simulink model "modeloNL1_HIL"  (R2025a)
settings: Solver=ode4  StartTime=0.0  StopTime=30  FixedStep=0.01  RelTol=1e-3
settings Model: Creator=anade  LastModifiedBy=Kaue

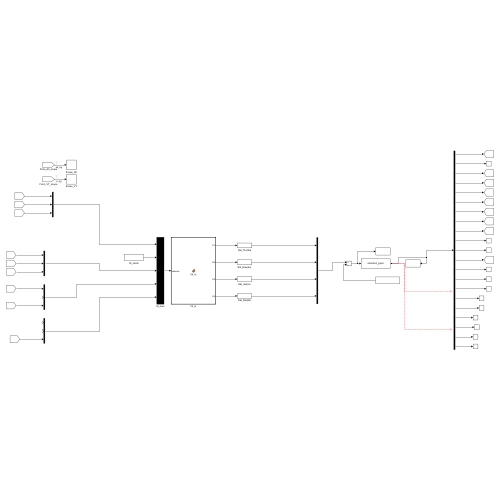
[thumbnail: Simulink's stored preview of the top-level diagram]
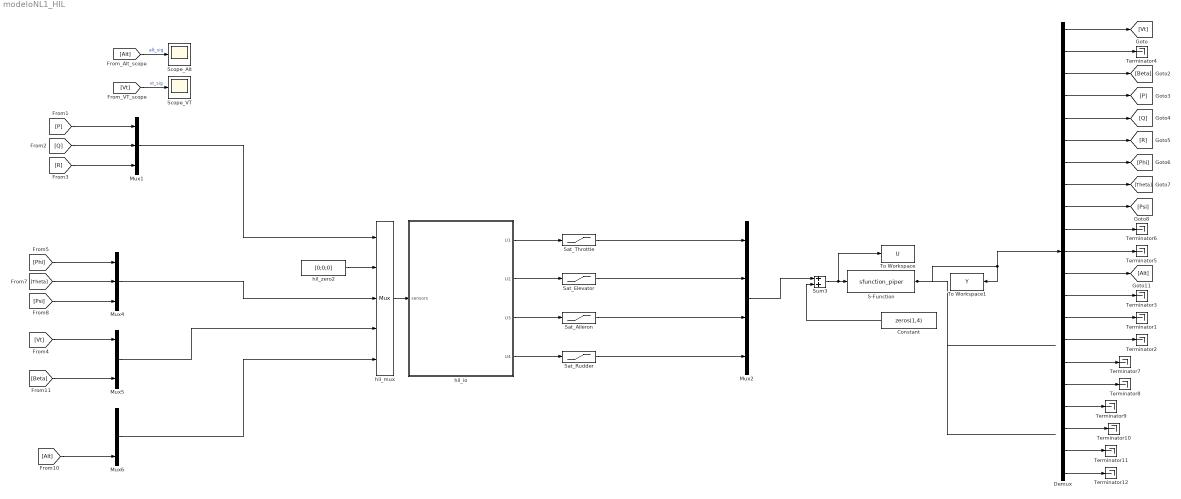
== system modeloNL1_HIL ==
  Constant : Constant  Value=zeros(1,4)
  Demux : Demux  Outputs=21
  Mux{1,4..6} (4 alike) : Mux  Inputs=3
  Mux2 : Mux
  S-Function : S-Function  FunctionName=sfunction_piper  Parameters=par_gen,par_aero,par_prop, Xe  SFunctionDeploymentMode=off  EnableBusSupport=off
  Sat_Aileron : Saturate  UpperLimit=0.4363  LowerLimit=-0.4363
  Sat_Elevator : Saturate  UpperLimit=0.4363  LowerLimit=-0.4363
  Sat_Rudder : Saturate  UpperLimit=0.4363  LowerLimit=-0.4363
  Sat_Throttle : Saturate  UpperLimit=1  LowerLimit=0
  Scope_Alt : Scope
      settings: ActiveDisplayYMinimum=80  ActiveDisplayYMaximum=120
  Scope_VT : Scope
      settings: ActiveDisplayYMinimum=10  ActiveDisplayYMaximum=20
  Sum3 : Sum
  Terminator{1..12} (12 alike) : Terminator
  To Workspace : ToWorkspace  VariableName=U  SaveFormat=Structure With Time  SampleTime=-1
  To Workspace1 : ToWorkspace  VariableName=Y  SaveFormat=Structure With Time  SampleTime=-1
  hil_io : MATLAB Function  TreatAsAtomicUnit=on
  hil_mux : Mux  Inputs=5
  hil_zero2 : Constant  Value=[0;0;0]
  wires:
  S-Function/1 -> To Workspace1/1, Demux/1
  Sum3/1 -> To Workspace/1, S-Function/1
  Mux2/1 -> Sum3/1
  Constant/1 -> Sum3/2
  Demux/2 -> Terminator4/1
  Demux/3 -> [Beta]
  Demux/4 -> [P]
  Demux/5 -> [Q]
  Demux/6 -> [R]
  Demux/7 -> [Phi]
  Demux/8 -> [Theta]
  Demux/10 -> Terminator6/1
  Demux/11 -> Terminator5/1
  Demux/13 -> Terminator3/1
  Demux/14 -> Terminator1/1
  Demux/15 -> Terminator2/1
  Demux/1 -> [Vt]
  [Theta] -> Mux4/2
  Mux1/1 -> hil_mux/1
  [Alt] -> Mux6/3
  [P] -> Mux1/1
  Mux4/1 -> hil_mux/3
  [R] -> Mux1/3
  [Phi] -> Mux4/1
  Mux6/1 -> hil_mux/5
  [Q] -> Mux1/2
  Mux5/1 -> hil_mux/4
  [Psi] -> Mux4/3
  [Beta] -> Mux5/3
  Demux/9 -> [Psi]
  [Vt] -> Mux5/1
  Demux/12 -> [Alt]
  Demux/17 -> Terminator8/1
  Demux/16 -> Terminator7/1
  Demux/19 -> Terminator10/1
  Demux/18 -> Terminator9/1
  Demux/21 -> Terminator12/1
  Demux/20 -> Terminator11/1
  Sat_Throttle/1 -> Mux2/1
  Sat_Elevator/1 -> Mux2/2
  Sat_Aileron/1 -> Mux2/3
  Sat_Rudder/1 -> Mux2/4
  hil_zero2/1 -> hil_mux/2
  hil_mux/1 -> hil_io/1(sensors)
  hil_io/1(U1) -> Sat_Throttle/1
  hil_io/2(U2) -> Sat_Elevator/1
  hil_io/3(U3) -> Sat_Aileron/1
  hil_io/4(U4) -> Sat_Rudder/1
  [Alt] -> Scope_Alt/1  "alt_sig"
  [Vt] -> Scope_VT/1  "vt_sig"

== matlab function modeloNL1_HIL/hil_io ==
  settings: updateMethod=DISCRETE  sampleTime=0.01
  data: sensors input double size=15; U1 output; U2 output; U3 output; U4 output
function [U1, U2, U3, U4] = hil_io(sensors)
%#codegen
U1 = 0; U2 = 0; U3 = 0; U4 = 0;
coder.extrinsic('hil_serial_step');
tmp = zeros(4,1);
tmp = hil_serial_step(sensors);
U1 = tmp(1);
U2 = tmp(2);
U3 = tmp(3);
U4 = tmp(4);
end
